simulink subsystem "Tracking_Regler_Side"  (R2023a)
settings: Solver=VariableStepAuto  StartTime=0.0  StopTime=10.0  RelTol=1e-3
undefined symbols (not defined in the file): F_int_side, G_side
settings Model: Creator=morit  LastModifiedBy=morit

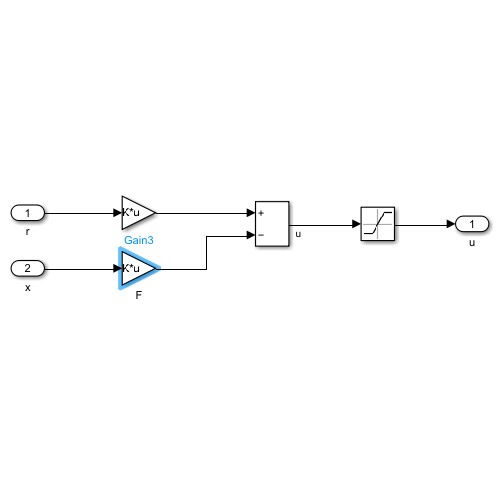
[thumbnail: Simulink's stored preview of the top-level diagram]
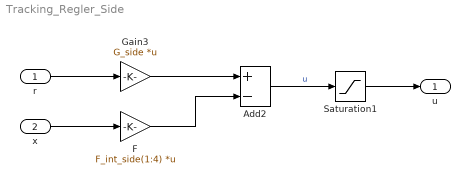
== system Tracking_Regler_Side ==
  r : Inport
  x : Inport  Port=2
  Add2 : Sum  Inputs=+-
  F : Gain  Gain=F_int_side(1:4)  Multiplication=Matrix(K*u)
  Gain3 : Gain  Gain=G_side  Multiplication=Matrix(K*u)
  Saturation1 : Saturate  UpperLimit=9  LowerLimit=-9
  u : Outport
  wires:
  r/1 -> Gain3/1
  Gain3/1 -> Add2/1
  Saturation1/1 -> u/1
  Add2/1 -> Saturation1/1  "u"
  F/1 -> Add2/2
  x/1 -> F/1
